simulink model "simulare"  (R2022a)
settings: Solver=VariableStepAuto  StartTime=0.0  StopTime=10.0  RelTol=1e-3
settings Model: Creator=saioc  LastModifiedBy=saioc

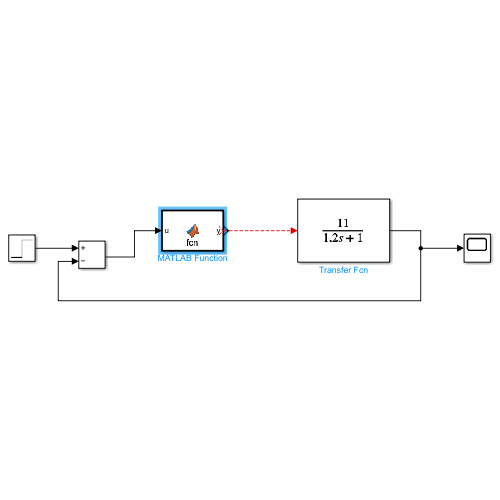
[thumbnail: Simulink's stored preview of the top-level diagram]
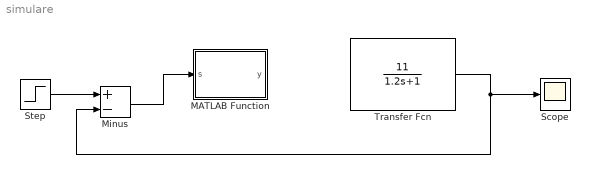
== system simulare ==
  MATLAB Function : MATLAB Function  TreatAsAtomicUnit=on
  Minus : Sum  Inputs=+-
  Scope : Scope
  Step : Step
  Transfer Fcn : TransferFcn  Numerator=[11]  Denominator=[1.2 1]
  wires:
  Transfer Fcn/1 -> Minus/2, Scope/1
  ? -> Transfer Fcn/1
  Step/1 -> Minus/1
  Minus/1 -> MATLAB Function/1(s)

== matlab function simulare/MATLAB Function ==
  data: s input; y output
function y = fcn(s)

y = (50*s^2 + 350*s + 300)/s;
